simulink model "quarter_car_model"  (R2021b)
settings: Solver=VariableStepAuto  StartTime=0.0  StopTime=5  RelTol=1e-3
values from neighbouring files (symbols this model uses):
  collisionTime = H/speed_ms    (= 0.012)    [quarter_car_sim.m]
  Cs = 2000    [quarter_car_sim.m]
  Ct = 0    [quarter_car_sim.m]
  freqR = 2*pi/interval_time    (= 8.72664625997)    [quarter_car_sim.m]
  Fsus = 0.0    (= 0)    [quarter_car_sim.m]
  gz = -9.81/6    (= -1.635)    [quarter_car_sim.m]
  H = 0.05    [quarter_car_sim.m]
  initial_shrink = (Mu+Ms)*abs(gz)/Kt    [quarter_car_sim.m]
  Ks = 40000    [quarter_car_sim.m]
  Kt = 200000    [quarter_car_sim.m]
  Ms = quarterMt*15.0/17.0    (= 1102.94117647)    [quarter_car_sim.m]
  Mu = quarterMt*2.0/17.0    (= 147.058823529)    [quarter_car_sim.m]
  rock = false    [quarter_car_sim.m]
libraries: simulink x1
settings Model: Creator=yuya onozuka  LastModifiedBy=yuya onozuka

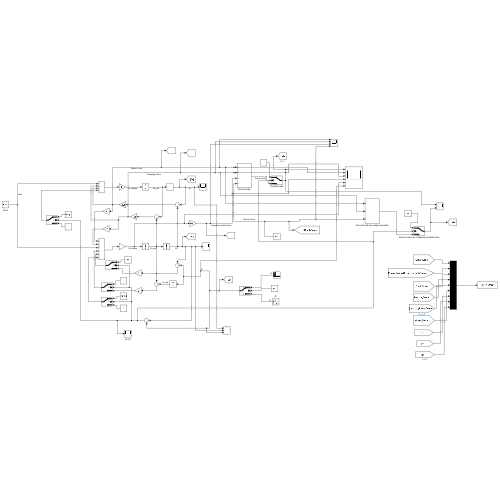
[thumbnail: Simulink's stored preview of the top-level diagram]
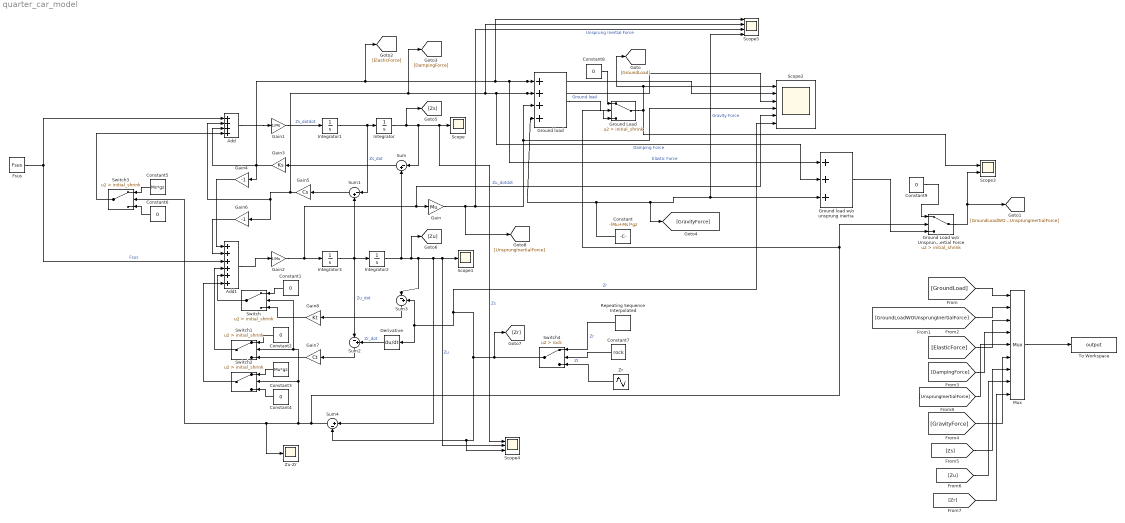
== system quarter_car_model ==
  Add : Sum  Inputs=++++
  Add1 : Sum  Inputs=++++++
  Constant : Constant  Value=-(Mu+Ms)*gz
  Constant{1..2,4,6,8..9} (6 alike) : Constant  Value=0
  Constant3 : Constant  Value=Mu*gz
  Constant5 : Constant  Value=Ms*gz
  Constant7 : Constant  Value=rock
  Derivative : Derivative
  Fsus : Constant  Value=Fsus
  Gain : Gain  Gain=Mu
  Gain1 : Gain  Gain=1/Ms
  Gain2 : Gain  Gain=1/Mu
  Gain3 : Gain  Gain=Ks
  Gain4 : Gain  Gain=-1
  Gain5 : Gain  Gain=Cs
  Gain6 : Gain  Gain=-1
  Gain7 : Gain  Gain=Ct
  Gain8 : Gain  Gain=Kt
  Ground Load : Switch  Criteria=u2 > Threshold  Threshold=initial_shrink
  Ground Load w/o Unsprung Inertial Force : Switch  Criteria=u2 > Threshold  Threshold=initial_shrink
  Ground load : Sum  Inputs=++++
  Ground load w/o unsprung inertia : Sum  Inputs=+++
  Integrator{,1..3} (4 alike) : Integrator
  Mux : Mux  Inputs=9
  Repeating Sequence Interpolated : simulink/Sources/Repeating Sequence Interpolated  OutValues=[0 0 H 0 0].'  TimeValues=[0 1 1+collisionTime 1+collisionTime*2 5].'  LookUpMeth=Interpolation-Use End Values  tsamp=0.01  OutMin=[]  OutMax=[]  OutDataTypeStr=double  OutputDataTypeScalingMode=double  OutDataType=fixdt(0,8)  OutScaling=2^-10
  Scope : Scope
  Scope1 : Scope
  Scope2 : Scope  NumInputPorts=6
  Scope3 : Scope  NumInputPorts=2
  Scope4 : Scope  NumInputPorts=3
  Scope5 : Scope  NumInputPorts=4
  Sum{,1..3} (4 alike) : Sum  Inputs=|-+
  Sum4 : Sum  Inputs=|+-
  Switch{,1..3} (4 alike) : Switch  Criteria=u2 > Threshold  Threshold=initial_shrink
  Switch4 : Switch  Criteria=u2 > Threshold  Threshold=rock
  To Workspace : ToWorkspace  VariableName=output  SaveFormat=Structure With Time  SampleTime=-1
  Zr : Sin  Amplitude=H/2  Bias=H/2  Frequency=freqR  Phase=3*pi/2  SampleTime=0
  Zu-Zr : Scope
  wires:
  Integrator/1 -> [Zs], Sum/1, Scope4/1, Scope/1  "Zs"
  Integrator1/1 -> Sum1/1, Integrator/1  "Zs_dot"
  Gain1/1 -> Integrator1/1  "Zs_dotdot"
  Add/1 -> Gain1/1
  Gain2/1 -> Scope2/5, Gain/1, Integrator3/1  "Zu_dotdot"
  Add1/1 -> Gain2/1
  Integrator3/1 -> Integrator2/1, Sum2/1, Sum1/2  "Zu_dot"
  Integrator2/1 -> [Zu], Sum3/1, Sum4/1, Scope4/2, Scope1/1, Sum/2  "Zu"
  Sum/1 -> Gain3/1
  Sum1/1 -> Gain5/1
  Gain5/1 -> [DampingForce], Scope5/2, Ground load w/o unsprung inertia/2, Scope2/3, Ground load/2, Add/2, Gain6/1  "Damping Force"
  Fsus/1 -> Add/1, Add1/3  "Fsus"
  Derivative/1 -> Sum2/2  "Zr_dot"
  Sum2/1 -> Gain7/1
  Sum3/1 -> Gain8/1
  Gain4/1 -> Add1/1
  Gain6/1 -> Add1/2
  Gain8/1 -> Switch/3
  Gain7/1 -> Switch1/3
  Constant/1 -> Ground load/4, [GravityForce], Scope5/4, Ground load w/o unsprung inertia/3  "Gravity Force"
  Ground load/1 -> Ground Load/3  "Ground load"
  Gain3/1 -> Scope5/1, Ground load w/o unsprung inertia/1, Scope2/2, Ground load/1, [ElasticForce], Add/3, Gain4/1  "Elastic Force"
  Gain/1 -> [UnsprungInertialForce], Scope5/3, Ground load/3, Scope2/4  "Unsprung Inertial Force"
  Switch4/1 -> [Zr], Scope4/3, Sum4/2, Derivative/1, Sum3/2, Scope2/6  "Zr"
  Constant1/1 -> Switch/1
  Switch/1 -> Add1/5
  Constant2/1 -> Switch1/1
  Switch1/1 -> Add1/4
  Constant3/1 -> Switch2/1
  Constant4/1 -> Switch2/3
  Switch2/1 -> Add1/6
  Constant5/1 -> Switch3/1
  Constant6/1 -> Switch3/3
  Switch3/1 -> Add/4
  Sum4/1 -> Ground Load w/o Unsprung Inertial Force/2, Ground Load/2, Switch/2, Switch1/2, Switch2/2, Zu-Zr/1, Switch3/2
  Zr/1 -> Switch4/3  "Zr"
  Repeating Sequence Interpolated/1 -> Switch4/1  "Zr"
  Constant7/1 -> Switch4/2
  Constant8/1 -> Ground Load/1
  Ground Load/1 -> Scope2/1, [GroundLoad], Scope3/1
  Constant9/1 -> Ground Load w/o Unsprung Inertial Force/1
  Ground load w/o unsprung inertia/1 -> Ground Load w/o Unsprung Inertial Force/3
  Ground Load w/o Unsprung Inertial Force/1 -> [GroundLoadWOUnsprungInertialForce], Scope3/2
  [GroundLoad] -> Mux/1
  [GroundLoadWOUnsprungInertialForce] -> Mux/2
  [ElasticForce] -> Mux/3
  [DampingForce] -> Mux/4
  [GravityForce] -> Mux/6
  [Zs] -> Mux/7
  [Zu] -> Mux/8
  [Zr] -> Mux/9
  Mux/1 -> To Workspace/1
  [UnsprungInertialForce] -> Mux/5
